simulink model "robot"  (R2016b)
settings: Solver=FixedStepDiscrete  StartTime=0.0  StopTime=inf  RelTol=1e-3
libraries: vexarmcortexlib x17
settings Model: ExtModeTrigDuration=25  Creator=Chase  LastModifiedBy=Chase
settings DataIOCC: LimitDataPoints=on  SignalLoggingSaveFormat=ModelDataLogs
settings OptimizationCC: DefaultParameterBehavior=Inlined  UseDivisionForNetSlopeComputation=on  UseFloatMulNetSlope=on  InlineInvariantSignals=on  PassReuseOutputArgsAs=Individual arguments  ExpressionDepthLimit=2147483647  ZeroExternalMemoryAtStartup=off  ZeroInternalMemoryAtStartup=off  NoFixptDivByZeroProtection=on  EfficientFloat2IntCast=on  LifeSpan=1  MaxStackSize=64
settings DebuggingCC: UnderspecifiedInitializationDetection=Classic  MergeDetectMultiDrivingBlocksExec=none  InheritedTsInSrcMsg=none  FcnCallInpInsideContextMsg=warning  UnconnectedInputMsg=none  UnconnectedOutputMsg=none  StateNameClashWarn=warning  SFUnexpectedBacktrackingDiag=warning  SFNoUnconditionalDefaultTransitionDiag=warning  SFExecutionAtInitializationDiag=none
settings HardwareCC: ProdBitPerPointer=32  ProdBitPerSizeT=32  ProdBitPerPtrDiffT=32  ProdLargestAtomicInteger=Long  ProdLargestAtomicFloat=Double  ProdIntDivRoundTo=Undefined  ProdWordSize=32  ProdHWDeviceType=ARM Compatible->ARM Cortex
settings ModelReferenceCC: PropagateSignalLabelsOutOfModel=off
settings RTWCC: SystemTargetFile=ert.tlc  HardwareBoard=ARM Cortex-based VEX Microcontroller  TemplateMakefile=ert_default_tmf  Description=Embedded Coder  GenerateReport=on  Toolchain=GNU Tools for VEX ARM Cortex  IncludeHyperlinkInReport=on  LaunchReport=on  TargetLang=C++  GenerateTraceInfo=on  GenerateTraceReport=on  GenerateTraceReportSl=on  GenerateTraceReportSf=on  GenerateTraceReportEml=on
settings CodeAppCC: ForceParamTrailComments=on  IgnoreCustomStorageClasses=off  SimulinkDataObjDesc=on  CustomSymbolStrGlobalVar=rt$N$M  CustomSymbolStrType=$N$M  CustomSymbolStrFcn=$N$M$F  CustomSymbolStrMacro=$N$M  InsertBlockDesc=on  InternalIdentifier=Classic
settings ERTTargetCC: TargetLangStandard=C++03 (ISO)  CodeReplacementLibrary=GCC ARM Cortex-M3  CombineSignalStateStructs=on  SupportAbsoluteTime=off  MultiInstanceERTCode=on  CodeInterfacePackaging=C++ class  SupportComplex=off  SupportNonInlinedSFcns=on  InlinedParameterPlacement=NonHierarchical  RootIOFormat=Structure reference  ERTFilePackagingFormat=CompactWithDataFile  ConvertIfToSwitch=off  SuppressUnreachableDefaultCases=off

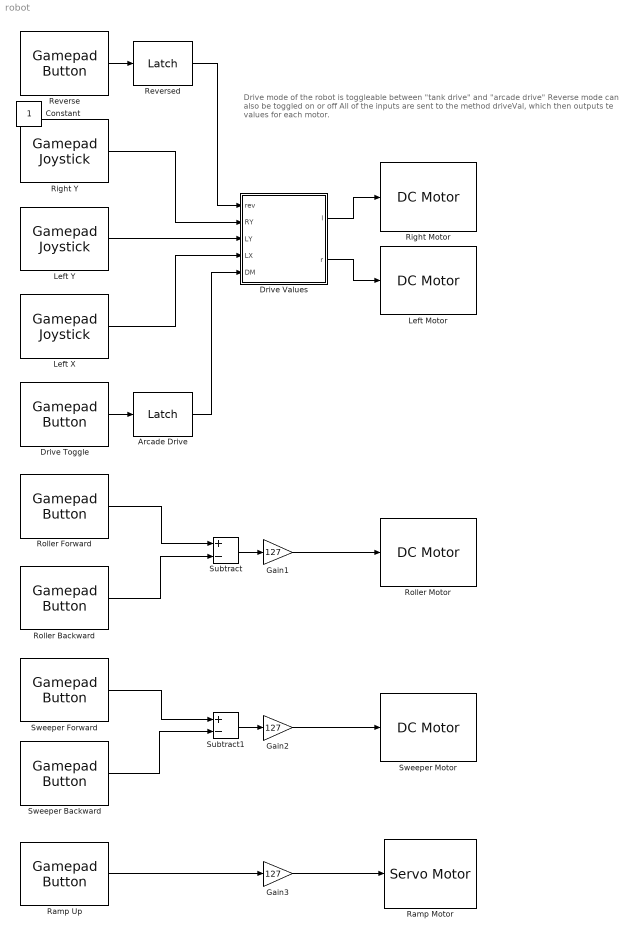
== system robot ==
  note: Drive mode of the robot is toggleable between "tank drive" and "arcade drive"
      |
      | Reverse mode can also be toggled on or off
      |
      | All of the inputs are sent to the method driveVal, which then outputs te values for each motor.
  Arcade Drive : vexarmcortexlib/Utilities/Latch  output0=off
  Drive Toggle : vexarmcortexlib/Gamepad Button  joystick=1  chan=6  button56=Up  button78=Right  SimulationIn=off  sample_time=0.2
  Drive Values : MATLAB Function  TreatAsAtomicUnit=on
      settings: CopyFcn=set_param(gcb, 'LinkStatus', 'none') ;
  Gain1 : Gain  Gain=127
  Gain2 : Gain  Gain=127
  Gain3 : Gain  Gain=127
  Left Motor : vexarmcortexlib/DC Motor  motor=3  scaleFactor=1/13.5  SimulationOut=off
  Left X : vexarmcortexlib/Gamepad Joystick  joystick=1  chan=4  SimulationIn=off  sample_time=0.2
  Left Y : vexarmcortexlib/Gamepad Joystick  joystick=1  chan=3  SimulationIn=off  sample_time=0.2
  Ramp Motor : vexarmcortexlib/Servo Motor  motor=6  scaleFactor=60/127  SimulationOut=off
  Ramp Up : vexarmcortexlib/Gamepad Button  joystick=1  chan=5  button56=Down  button78=Right  SimulationIn=off  sample_time=0.2
  Reverse : vexarmcortexlib/Gamepad Button  joystick=1  chan=5  button56=Up  button78=Right  SimulationIn=off  sample_time=0.2
  Reversed : vexarmcortexlib/Utilities/Latch  output0=off
  Right Motor : vexarmcortexlib/DC Motor  motor=2  scaleFactor=1/13.5  SimulationOut=off
  Right Y : vexarmcortexlib/Gamepad Joystick  joystick=1  chan=2  SimulationIn=off  sample_time=0.2
  Roller Backward : vexarmcortexlib/Gamepad Button  joystick=1  chan=7  button56=Up  button78=Down  SimulationIn=off  sample_time=0.2
  Roller Forward : vexarmcortexlib/Gamepad Button  joystick=1  chan=7  button56=Up  button78=Up  SimulationIn=off  sample_time=0.2
  Roller Motor : vexarmcortexlib/DC Motor  motor=3  scaleFactor=1/13.5  SimulationOut=off
  Subtract : Sum  Inputs=+-
  Subtract1 : Sum  Inputs=+-
  Sweeper Backward : vexarmcortexlib/Gamepad Button  joystick=1  chan=8  button56=Up  button78=Down  SimulationIn=off  sample_time=0.2
  Sweeper Forward : vexarmcortexlib/Gamepad Button  joystick=1  chan=8  button56=Up  button78=Up  SimulationIn=off  sample_time=0.2
  Sweeper Motor : vexarmcortexlib/DC Motor  motor=5  scaleFactor=1/13.5  SimulationOut=off
  Constant : Constant  IOType=siggen
  wires:
  Reverse/1 -> Reversed/1
  Drive Toggle/1 -> Arcade Drive/1
  Roller Forward/1 -> Subtract/1
  Roller Backward/1 -> Subtract/2
  Subtract/1 -> Gain1/1
  Gain1/1 -> Roller Motor/1
  Subtract1/1 -> Gain2/1
  Sweeper Forward/1 -> Subtract1/1
  Sweeper Backward/1 -> Subtract1/2
  Gain2/1 -> Sweeper Motor/1
  Left Y/1 -> Drive Values/3(LY)
  Left X/1 -> Drive Values/4(LX)
  Arcade Drive/1 -> Drive Values/5(DM)
  Right Y/1 -> Drive Values/2(RY)
  Reversed/1 -> Drive Values/1(rev)
  Drive Values/2(r) -> Left Motor/1
  Drive Values/1(l) -> Right Motor/1
  Ramp Up/1 -> Gain3/1
  Gain3/1 -> Ramp Motor/1

== matlab function robot/Drive Values ==
  data: rev input; l output; RY input; LY input; LX input; DM input; r output
function [l, r] = driveVal(rev, RY, LY, LX, DM)
    %# Before this if, rev is a boolean value
    %# After this if, rev becomes the reverseDM modifier
    if rev == 1 
        rev = -1;   %# If the robot is reversed, change its modifier to reflect
    else
        rev = 1;    %# If the robot is not reversed, change its modifier to reflect
    end
    
    if DM == 1   %# Drive mode is Arcade
        l = (RY + LX) * rev;
        r = (RY - LX) * rev;
    else        %# Drive mode is Tank
        l = LY * rev;
        r = RY * rev;
    end
end
